simulink model "NPNwithVVI_2018a"  (R2018a)
settings: Solver=FixedStepDiscrete  StartTime=0.0  StopTime=10000  FixedStep=1  RelTol=1e-3  EnableMultiTasking=on
libraries: model_library x1
settings Model: SnapshotInterval=1  Creator=houssamabbas  LastModifiedBy=aronharder
settings SolverCC: AutoInsertRateTranBlk=on
settings OptimizationCC: LifeSpan=inf
settings DebuggingCC: SFUnexpectedBacktrackingDiag=warning  SFNoUnconditionalDefaultTransitionDiag=warning  SFExecutionAtInitializationDiag=none
settings CodeAppCC: StateflowObjectComments=on
settings GRTTargetCC: TargetLangStandard=C89/C90 (ANSI)
settings ConfigComp: CovMetricSettings=dw  CovHtmlReporting=on  CovSaveCumulativeToWorkspaceVar=on  CovSaveSingleToWorkspaceVar=on  CovExternalEMLEnable=off

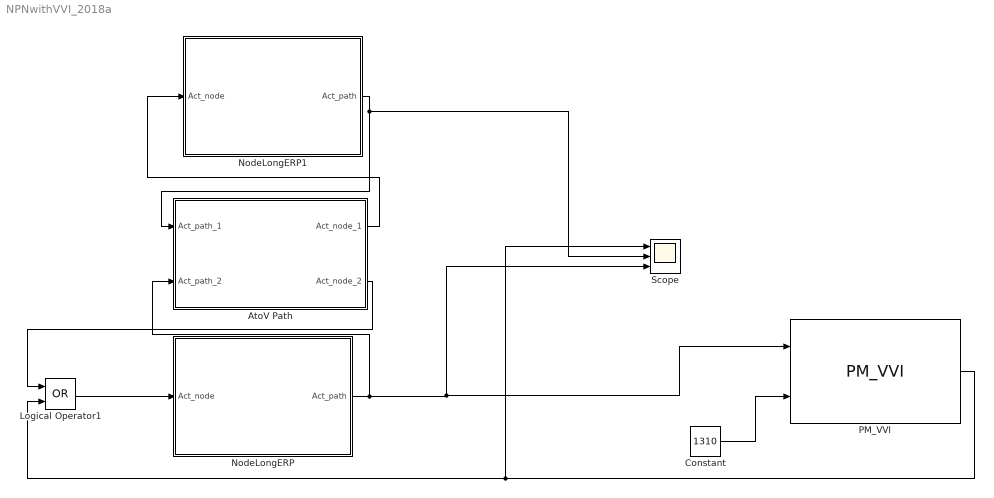
== system NPNwithVVI_2018a ==
  AtoV Path : Subsystem  AncestorBlock=model_library/Path_a2
  Constant : Constant  Value=1310  OutDataTypeStr=uint16
  Logical Operator1 : Logic  Operator=OR  AllPortsSameDT=off  OutDataTypeStr=boolean
  NodeLongERP : Subsystem  AncestorBlock=model_library/Node_a2
  NodeLongERP1 : Subsystem  AncestorBlock=model_library/Node_a2
  PM_VVI : model_library/PM_VVI  SystemSampleTime=-1
  Scope : Scope  NumInputPorts=3
  wires:
  NodeLongERP1/1(Act_path) -> Scope/2, AtoV Path/1(Act_path_1)
  AtoV Path/2(Act_node_2) -> Logical Operator1/1
  NodeLongERP/1(Act_path) -> PM_VVI/1, Scope/3, AtoV Path/2(Act_path_2)
  AtoV Path/1(Act_node_1) -> NodeLongERP1/1(Act_node)
  Logical Operator1/1 -> NodeLongERP/1(Act_node)
  PM_VVI/1 -> Scope/1, Logical Operator1/2
  Constant/1 -> PM_VVI/2

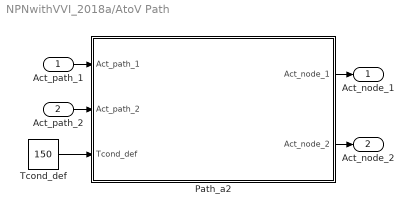
== system NPNwithVVI_2018a/AtoV Path ==
  Act_path_1 : Inport
  Act_path_2 : Inport  Port=2
  Path_a2 : Stateflow chart  TreatAsAtomicUnit=on
  Tcond_def : Constant  Value=150  OutDataTypeStr=uint16
  Act_node_1 : Outport
  Act_node_2 : Outport  Port=2
  wires:
  Tcond_def/1 -> Path_a2/3(Tcond_def)
  Path_a2/2(Act_node_2) -> Act_node_2/1
  Act_path_1/1 -> Path_a2/1(Act_path_1)
  Act_path_2/1 -> Path_a2/2(Act_path_2)
  Path_a2/1(Act_node_1) -> Act_node_1/1

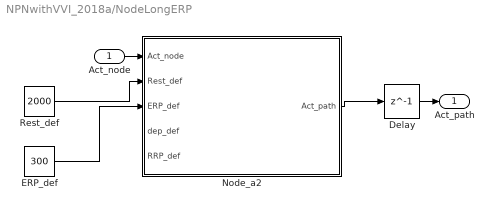
== system NPNwithVVI_2018a/NodeLongERP ==
  Act_node : Inport
  Delay : Delay  DelayLength=1  InitialCondition=0
  ERP_def : Constant  Value=300  OutDataTypeStr=uint16
  Node_a2 : Stateflow chart  RequirementInfo="{}  %GIDa_6ee29377_7781_44c0_ad76_b00d26592997"  TreatAsAtomicUnit=on
  Rest_def : Constant  Value=2000  OutDataTypeStr=uint16
  Act_path : Outport
  wires:
  Delay/1 -> Act_path/1
  ERP_def/1 -> Node_a2/3(ERP_def)
  Rest_def/1 -> Node_a2/2(Rest_def)
  Act_node/1 -> Node_a2/1(Act_node)
  Node_a2/1(Act_path) -> Delay/1

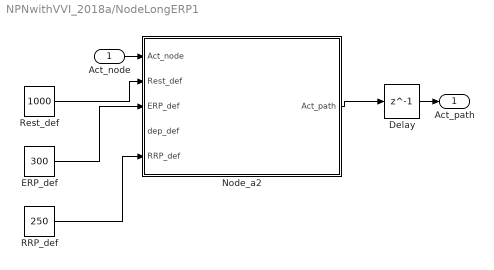
== system NPNwithVVI_2018a/NodeLongERP1 ==
  Act_node : Inport
  Delay : Delay  DelayLength=1  InitialCondition=0
  ERP_def : Constant  Value=300  OutDataTypeStr=uint16
  Node_a2 : Stateflow chart  RequirementInfo="{}  %GIDa_6ee29377_7781_44c0_ad76_b00d26592997"  TreatAsAtomicUnit=on
  RRP_def : Constant  Value=250  OutDataTypeStr=uint16
  Rest_def : Constant  Value=1000  OutDataTypeStr=uint16
  Act_path : Outport
  wires:
  Delay/1 -> Act_path/1
  ERP_def/1 -> Node_a2/3(ERP_def)
  Rest_def/1 -> Node_a2/2(Rest_def)
  Act_node/1 -> Node_a2/1(Act_node)
  Node_a2/1(Act_path) -> Delay/1
  RRP_def/1 -> Node_a2/5(RRP_def)

== stateflow chart NPNwithVVI_2018a/NodeLongERP/Node_a2 ==
  state node
    settings: description=|
        | temp can be thought of a sub-mode of ERP, which only exists to make sure that act_path is high for one period.
        | 
        | In ERP, if Act_node is received, then it is ignored through that self-transition.
        | 
        | Note this doesn't model variations in cycle length because everytime it is stimulated in RRP, ERP_cur is set to ERP_def again.
    state Rest
    state RRP
    state ERP
    state temp
    (default) -> Rest : {Rest_cur=Rest_def;}
    Rest -> temp [order 3] : [Act_node==false && Rest_cur<=uint16(0)]/{Act_path=true;uptime= uint16(0);ERP_cur=ERP_def;}
    Rest -> temp [order 1] : [Act_node==true]/{Act_path=true;uptime= uint16(0);ERP_cur=ERP_def;}
    Rest -> Rest [order 2] : [Act_node==false && Rest_cur>uint16(0)]/{Rest_cur = Rest_cur - uint16(1);}
    RRP -> Rest [order 1] : [RRP_cur<=0]/{Rest_cur=Rest_def;}
    RRP -> RRP [order 2] : [Act_node==false && RRP_cur>0]/{RRP_cur=RRP_cur-uint16(1);}
    RRP -> temp [order 3] : [Act_node==true]/{Act_path=true;uptime= uint16(0);ERP_cur=ERP_def;}
    ERP -> RRP [order 1] : [ERP_cur<=uint16(0)]/{RRP_cur=RRP_def;}
    temp -> temp [order 1] : [uptime<uint16(1)]/{uptime = uptime + uint16(1);ERP_cur =ERP_cur - uint16(1);}
    temp -> ERP [order 2] : [uptime>=uint16(1)]/{Act_path=false;}
    ERP -> ERP [order 3] : [Act_node==true]
    ERP -> ERP [order 2] : {ERP_cur = ERP_cur - uint16(1);}
  data: Act_node input boolean; Act_path output boolean; Rest_cur local uint16; ERP_cur local uint16; Rest_def input uint16; ERP_def input uint16; uptime local uint16; dep_cur local uint16; dep_def input uint16; RRP_cur local uint16; RRP_def input uint16

== stateflow chart NPNwithVVI_2018a/NodeLongERP1/Node_a2 ==
  state node
    settings: description=|
        | temp can be thought of a sub-mode of ERP, which only exists to make sure that act_path is high for one period.
        | 
        | In ERP, if Act_node is received, then it is ignored through that self-transition.
        | 
        | Note this doesn't model variations in cycle length because everytime it is stimulated in RRP, ERP_cur is set to ERP_def again.
    state Rest
    state RRP
    state ERP
    state temp
    (default) -> Rest : {Rest_cur=Rest_def;}
    Rest -> temp [order 3] : [Act_node==false && Rest_cur<=uint16(0)]/{Act_path=true;uptime= uint16(0);ERP_cur=ERP_def;}
    Rest -> temp [order 1] : [Act_node==true]/{Act_path=true;uptime= uint16(0);ERP_cur=ERP_def;}
    Rest -> Rest [order 2] : [Act_node==false && Rest_cur>uint16(0)]/{Rest_cur = Rest_cur - uint16(1);}
    RRP -> Rest [order 1] : [RRP_cur<=0]/{Rest_cur=Rest_def;}
    RRP -> RRP [order 2] : [Act_node==false && RRP_cur>0]/{RRP_cur=RRP_cur-uint16(1);}
    RRP -> temp [order 3] : [Act_node==true]/{Act_path=true;uptime= uint16(0);ERP_cur=ERP_def;}
    ERP -> RRP [order 1] : [ERP_cur<=uint16(0)]/{RRP_cur=RRP_def;}
    temp -> temp [order 1] : [uptime<uint16(1)]/{uptime = uptime + uint16(1);ERP_cur =ERP_cur - uint16(1);}
    temp -> ERP [order 2] : [uptime>=uint16(1)]/{Act_path=false;}
    ERP -> ERP [order 3] : [Act_node==true]
    ERP -> ERP [order 2] : {ERP_cur = ERP_cur - uint16(1);}
  data: Act_node input boolean; Act_path output boolean; Rest_cur local uint16; ERP_cur local uint16; Rest_def input uint16; ERP_def input uint16; uptime local uint16; dep_cur local uint16; dep_def input uint16; RRP_cur local uint16; RRP_def input uint16

== stateflow chart NPNwithVVI_2018a/AtoV Path/Path_a2 ==
  state path
    state Idle
    state Ante
    state Retro
    state Conflict
    state Double
    (default) -> Idle
    Idle -> Ante [order 1] : [Act_path_1==true]/{Tcond_cur=Tcond_def;}
    Idle -> Retro [order 2] : [Act_path_2==true]/{Tcond_cur=Tcond_def;}
    Conflict -> Idle [order 1] : [uptime>0]/{Act_node_1=false;Act_node_2=false;}
    Ante -> Ante [order 3] : [Act_path_2==false && Tcond_cur>uint16(0)]/{Tcond_cur = Tcond_cur - uint16(1);}
    Retro -> Retro [order 3] : [Act_path_1==false && Tcond_cur>uint16(0)]/{Tcond_cur = Tcond_cur - uint16(1);}
    Ante -> Double [order 2] : [Act_path_2==true]
    Ante -> Conflict [order 1] : [Act_path_2==false && Tcond_cur<=uint16(0)]/{Act_node_2=true;uptime=uint16(0);}
    Retro -> Conflict [order 1] : [Act_path_1==false && Tcond_cur<=uint16(0)]/{Act_node_1=true;uptime=uint16(0);}
    Retro -> Double [order 2] : [Act_path_1==true]
    Conflict -> Conflict [order 2] : [uptime<=uint16(0)]/{uptime = uptime + uint16(1);}
    Double -> Conflict : [Tcond_cur<=uint16(0)]/{uptime=uint16(0);}
  data: Act_path_1 input boolean; Act_path_2 input boolean; Act_node_1 output boolean; Act_node_2 output boolean; Tcond_cur local uint16; Tcond_def input uint16; uptime local uint16
